simulink model "RC_circuit"  (R2024b)
settings: Solver=VariableStepAuto  StartTime=0.0  StopTime=10.0  RelTol=1e-3
settings Model: Creator=Utilizador  LastModifiedBy=Utilizador

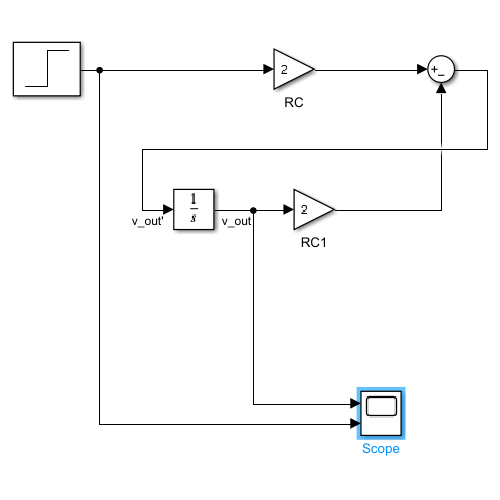
[thumbnail: Simulink's stored preview of the top-level diagram]
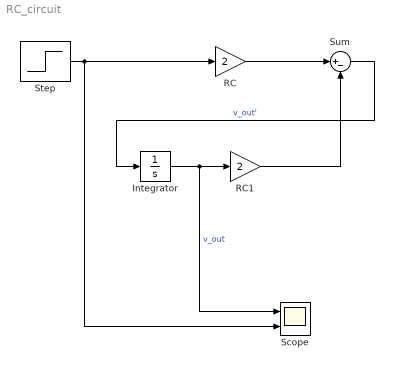
== system RC_circuit ==
  Integrator : Integrator
  RC : Gain  Gain=2
  RC1 : Gain  Gain=2
  Scope : Scope  NumInputPorts=2
  Step : Step  After=5  SampleTime=0
  Sum : Sum  Inputs=|+-
  wires:
  Sum/1 -> Integrator/1  "v_out'"
  Integrator/1 -> RC1/1, Scope/1  "v_out"
  Step/1 -> RC/1, Scope/2
  RC1/1 -> Sum/2
  RC/1 -> Sum/1
